simulink model "V511_L2"  (R2023b)
settings: Solver=FixedStepAuto  StartTime=0.0  StopTime=10  FixedStep=1  MaxStep=0.01  RelTol=1e-3
libraries: simulink x15
settings Model: Creator=td  LastModifiedBy=killer
settings SolverCC: AlgebraicLoopSolver=TrustRegion
settings DataIOCC: ReturnWorkspaceOutputs=off
settings DebuggingCC: UnconnectedInputMsg=warning  UnconnectedOutputMsg=warning  UnconnectedLineMsg=warning  ArithmeticOperatorsInVariantConditions=warning
settings ModelReferenceCC: EnableRefExpFcnMdlSchedulingChecks=on
settings SFSimCC: CustomCodeUndefinedFunction=UseInterfaceOnly

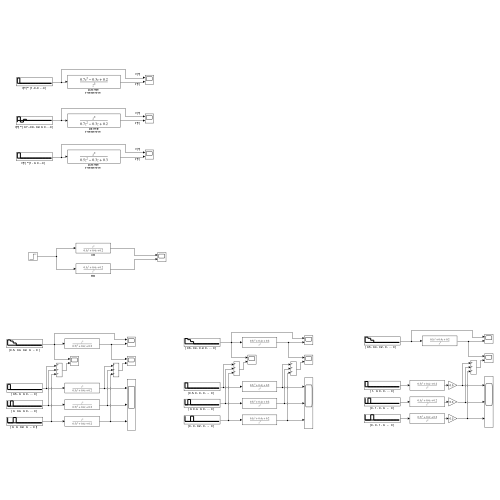
[thumbnail: Simulink's stored preview of the top-level diagram]
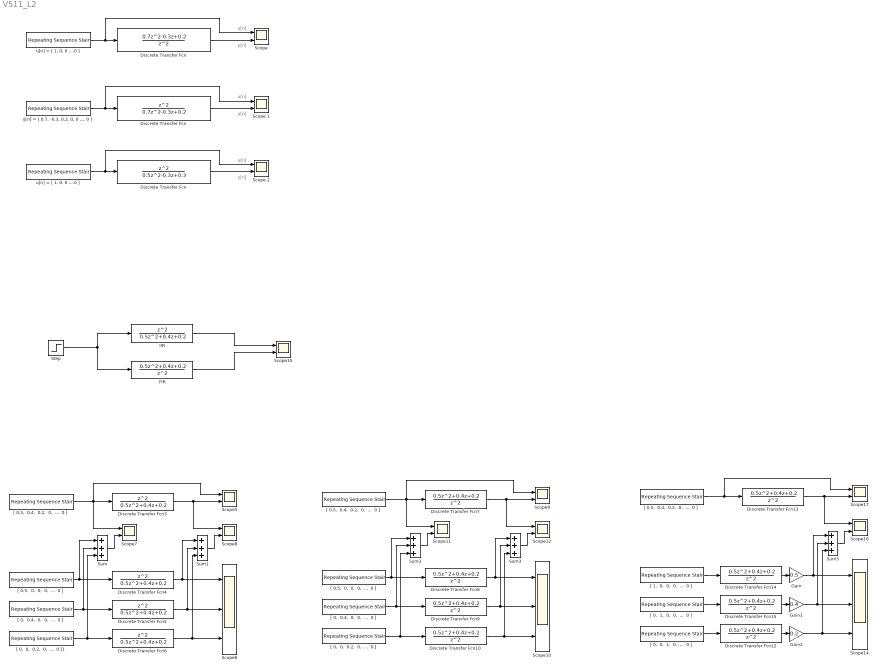
== system V511_L2 ==
  note: u[n]
  note: y[n]
  note: u[n]
  note: y[n]
  note: u[n]
  note: y[n]
  " Discrete Transfer Fcn " : DiscreteTransferFcn  Numerator=[1 0 0]  Denominator=[0.7 -0.3 0.2]  SampleTime=1
  " [ 0,  0,  1,  0,  ...  0 ] " : simulink/Sources/Repeating Sequence Stair  OutValues="[0 0 1 0 0 0  0 0 0 0 0 0]"  tsamp=1  OutMin=[]  OutMax=[]  OutDataTypeStr=double  OutputDataTypeScalingMode=double  OutDataType=fixdt(0,8)  ConRadixGroup=Best Precision: Vector-wise  OutScaling=2^-12
  " [ 0,  1,  0,  0,  ...  0 ] " : simulink/Sources/Repeating Sequence Stair  OutValues="[0 1 0 0 0 0  0 0 0 0 0 0]"  tsamp=1  OutMin=[]  OutMax=[]  OutDataTypeStr=double  OutputDataTypeScalingMode=double  OutDataType=fixdt(0,8)  ConRadixGroup=Best Precision: Vector-wise  OutScaling=2^-12
  " [ 1,  0,  0,  0,  ...  0 ]" : simulink/Sources/Repeating Sequence Stair  OutValues="[1 0 0 0 0 0  0 0 0 0 0 0]"  tsamp=1  OutMin=[]  OutMax=[]  OutDataTypeStr=double  OutputDataTypeScalingMode=double  OutDataType=fixdt(0,8)  ConRadixGroup=Best Precision: Vector-wise  OutScaling=2^-12
  "Discrete Transfer Fcn   " : DiscreteTransferFcn  Numerator=[1 0 0]  Denominator=[0.5 -0.3 0.3]  SampleTime=1
  "Discrete Transfer Fcn " : DiscreteTransferFcn  Numerator=[0.7 -0.3 0.2]  Denominator=[1 0 0]  SampleTime=1
  Discrete Transfer Fcn{7..10,12..15} (8 alike) : DiscreteTransferFcn  Numerator=[0.5 0.4 0.2]  Denominator=[1 0 0]
  Discrete Transfer Fcn{3..6} (4 alike) : DiscreteTransferFcn  Numerator="[1 0 0  ]"  Denominator=[0.5 0.4 0.2]
  FIR : DiscreteTransferFcn  Numerator=[0.5 0.4 0.2]  Denominator=[1 0 0]
  Gain : Gain  Gain=0.5
  Gain1 : Gain  Gain=0.4
  Gain2 : Gain  Gain=0.2
  IIR : DiscreteTransferFcn  Numerator=[1 0 0 ]  Denominator=[0.5 0.4 0.2]
  "Scope " : Scope  NumInputPorts=2
  Scope 1 : Scope  NumInputPorts=2
  Scope 2 : Scope  NumInputPorts=2
  Scope10 : Scope  NumInputPorts=3
  Scope{5,7..9,11..12,15..17} (9 alike) : Scope  NumInputPorts=2
  Scope14 : Scope  NumInputPorts=3
  Scope6 : Scope  NumInputPorts=3
  Step : Step  Time=0  SampleTime=0
  Sum{,1..3,5} (5 alike) : Sum  Inputs=+++
  "[ 0,  0,  0.2,  0,  ...  0 ]  " : simulink/Sources/Repeating Sequence Stair  OutValues="[0 0 0.2 0 0 0  0 0 0 0 0 0]"  tsamp=1  OutMin=[]  OutMax=[]  OutDataTypeStr=double  OutputDataTypeScalingMode=double  OutDataType=fixdt(0,8)  ConRadixGroup=Best Precision: Vector-wise  OutScaling=2^-12
  "[ 0,  0,  0.2,  0,  ...  0 ]1" : simulink/Sources/Repeating Sequence Stair  OutValues="[0 0 0.2 0 0 0  0 0 0 0 0 0]"  tsamp=1  OutMin=[]  OutMax=[]  OutDataTypeStr=double  OutputDataTypeScalingMode=double  OutDataType=fixdt(0,8)  ConRadixGroup=Best Precision: Vector-wise  OutScaling=2^-12
  "[ 0,  0.4,  0,  0,  ...  0 ]" : simulink/Sources/Repeating Sequence Stair  OutValues="[0 0.4 0 0 0 0  0 0 0 0 0 0]"  tsamp=1  OutMin=[]  OutMax=[]  OutDataTypeStr=double  OutputDataTypeScalingMode=double  OutDataType=fixdt(0,8)  ConRadixGroup=Best Precision: Vector-wise  OutScaling=2^-12
  "[ 0,  0.4,  0,  0,  ...  0 ] " : simulink/Sources/Repeating Sequence Stair  OutValues="[0 0.4 0 0 0 0  0 0 0 0 0 0]"  tsamp=1  OutMin=[]  OutMax=[]  OutDataTypeStr=double  OutputDataTypeScalingMode=double  OutDataType=fixdt(0,8)  ConRadixGroup=Best Precision: Vector-wise  OutScaling=2^-12
  "[ 0.5,  0,  0,  0,  ...  0 ]" : simulink/Sources/Repeating Sequence Stair  OutValues="[0.5 0 0 0 0 0  0 0 0 0 0 0]"  tsamp=1  OutMin=[]  OutMax=[]  OutDataTypeStr=double  OutputDataTypeScalingMode=double  OutDataType=fixdt(0,8)  ConRadixGroup=Best Precision: Vector-wise  OutScaling=2^-12
  "[ 0.5,  0,  0,  0,  ...  0 ]  " : simulink/Sources/Repeating Sequence Stair  OutValues="[0.5 0 0 0 0 0  0 0 0 0 0 0]"  tsamp=1  OutMin=[]  OutMax=[]  OutDataTypeStr=double  OutputDataTypeScalingMode=double  OutDataType=fixdt(0,8)  ConRadixGroup=Best Precision: Vector-wise  OutScaling=2^-12
  "[ 0.5,  0.4,  0.2,  0,  ...  0 ]" : simulink/Sources/Repeating Sequence Stair  OutValues="[0.5 0.4 0.2 0 0 0  0 0 0 0 0 0]"  tsamp=1  OutMin=[]  OutMax=[]  OutDataTypeStr=double  OutputDataTypeScalingMode=double  OutDataType=fixdt(0,8)  ConRadixGroup=Best Precision: Vector-wise  OutScaling=2^-12
  "[ 0.5,  0.4,  0.2,  0,  ...  0 ]  " : simulink/Sources/Repeating Sequence Stair  OutValues="[0.5 0.4 0.2 0 0 0  0 0 0 0 0 0]"  tsamp=1  OutMin=[]  OutMax=[]  OutDataTypeStr=double  OutputDataTypeScalingMode=double  OutDataType=fixdt(0,8)  ConRadixGroup=Best Precision: Vector-wise  OutScaling=2^-12
  "[ 0.5,  0.4,  0.2,  0,  ...  0 ]   " : simulink/Sources/Repeating Sequence Stair  OutValues="[0.5 0.4 0.2 0 0 0  0 0 0 0 0 0]"  tsamp=1  OutMin=[]  OutMax=[]  OutDataTypeStr=double  OutputDataTypeScalingMode=double  OutDataType=fixdt(0,8)  ConRadixGroup=Best Precision: Vector-wise  OutScaling=2^-12
  "u[n] = [ 0.7, -0.3, 0.2, 0, 0 .... 0 ]" : simulink/Sources/Repeating Sequence Stair  OutValues="[0.7 -0.3 0.2 0 0 0  0 0 0 0 0]"  tsamp=1  OutMin=[]  OutMax=[]  OutDataTypeStr=double  OutputDataTypeScalingMode=double  OutDataType=fixdt(0,8)  ConRadixGroup=Best Precision: Vector-wise  OutScaling=2^-12
  "u[n] = [ 1, 0, 0 ....0 ]" : simulink/Sources/Repeating Sequence Stair  OutValues=[1 0 0 0 0 0 0 0 0 0 0 0 0]  tsamp=1  OutMin=[]  OutMax=[]  OutDataTypeStr=double  OutputDataTypeScalingMode=double  OutDataType=fixdt(0,8)  ConRadixGroup=Best Precision: Vector-wise  OutScaling=2^-12
  "u[n] = [ 1, 0, 0 ....0 ]  " : simulink/Sources/Repeating Sequence Stair  OutValues="[1 0 0 0 0 0  0 0 0 0 0]"  tsamp=1  OutMin=[]  OutMax=[]  OutDataTypeStr=double  OutputDataTypeScalingMode=double  OutDataType=fixdt(0,8)  ConRadixGroup=Best Precision: Vector-wise  OutScaling=2^-12
  wires:
  "[ 0.5,  0.4,  0.2,  0,  ...  0 ]"/1 -> Discrete Transfer Fcn3/1, Scope5/1, Scope7/1
  Discrete Transfer Fcn3/1 -> Scope8/1, Scope5/2
  Discrete Transfer Fcn4/1 -> Scope6/1, Sum1/1
  Discrete Transfer Fcn5/1 -> Scope6/2, Sum1/2
  Discrete Transfer Fcn6/1 -> Scope6/3, Sum1/3
  "[ 0,  0,  0.2,  0,  ...  0 ]1"/1 -> Discrete Transfer Fcn6/1, Sum/3
  "[ 0,  0.4,  0,  0,  ...  0 ]"/1 -> Discrete Transfer Fcn5/1, Sum/2
  "[ 0.5,  0,  0,  0,  ...  0 ]"/1 -> Sum/1, Discrete Transfer Fcn4/1
  Sum/1 -> Scope7/2
  Sum1/1 -> Scope8/2
  "Discrete Transfer Fcn "/1 -> "Scope "/2
  "u[n] = [ 1, 0, 0 ....0 ]"/1 -> "Scope "/1, "Discrete Transfer Fcn "/1
  Sum2/1 -> Scope11/2
  Sum3/1 -> Scope12/2
  Discrete Transfer Fcn9/1 -> Scope10/2, Sum3/2
  Discrete Transfer Fcn10/1 -> Scope10/3, Sum3/3
  "[ 0,  0,  0.2,  0,  ...  0 ]  "/1 -> Discrete Transfer Fcn10/1, Sum2/3
  "[ 0,  0.4,  0,  0,  ...  0 ] "/1 -> Discrete Transfer Fcn9/1, Sum2/2
  "[ 0.5,  0,  0,  0,  ...  0 ]  "/1 -> Sum2/1, Discrete Transfer Fcn8/1
  Discrete Transfer Fcn7/1 -> Scope12/1, Scope9/2
  Discrete Transfer Fcn8/1 -> Scope10/1, Sum3/1
  "[ 0.5,  0.4,  0.2,  0,  ...  0 ]  "/1 -> Discrete Transfer Fcn7/1, Scope9/1, Scope11/1
  " [ 0,  1,  0,  0,  ...  0 ] "/1 -> Discrete Transfer Fcn15/1
  " [ 1,  0,  0,  0,  ...  0 ]"/1 -> Discrete Transfer Fcn14/1
  Gain1/1 -> Scope14/2, Sum5/2
  " [ 0,  0,  1,  0,  ...  0 ] "/1 -> Discrete Transfer Fcn12/1
  Discrete Transfer Fcn13/1 -> Scope16/1, Scope17/2
  Gain2/1 -> Scope14/3, Sum5/3
  Sum5/1 -> Scope16/2
  Gain/1 -> Scope14/1, Sum5/1
  "[ 0.5,  0.4,  0.2,  0,  ...  0 ]   "/1 -> Discrete Transfer Fcn13/1, Scope17/1
  Discrete Transfer Fcn14/1 -> Gain/1
  Discrete Transfer Fcn15/1 -> Gain1/1
  Discrete Transfer Fcn12/1 -> Gain2/1
  Step/1 -> FIR/1, IIR/1
  IIR/1 -> Scope15/1
  FIR/1 -> Scope15/2
  " Discrete Transfer Fcn "/1 -> Scope 1/2
  "u[n] = [ 0.7, -0.3, 0.2, 0, 0 .... 0 ]"/1 -> Scope 1/1, " Discrete Transfer Fcn "/1
  "Discrete Transfer Fcn   "/1 -> Scope 2/2
  "u[n] = [ 1, 0, 0 ....0 ]  "/1 -> Scope 2/1, "Discrete Transfer Fcn   "/1
